simulink model "simpleObserver2withKalman"  (R2021b)
settings: Solver=ode1  StartTime=0.0  StopTime=inf  FixedStep=0.01  RelTol=1e-3
libraries: TcTargetLib x10
settings Model: Creator=ATLabor  LastModifiedBy=ATLabor
settings OptimizationCC: DefaultParameterBehavior=Inlined  LocalBlockOutputs=off
settings RTWCC: Description=TwinCAT GRT Target  SystemTargetFile=TwinCatGrt.tlc  GenCodeOnly=on  TemplateMakefile=tcgrt_msbuild.tmf  TargetLang=C++
settings STFCustomTargetCC: TargetLangStandard=C++11 (ISO)  CombineOutputUpdateFcns=on  CodeInterfacePackaging=Reusable function  CPPClassGenCompliant=on  GRTInterface=off  GenerateAllocFcn=on  SystemTargetFile=TwinCatGrt.tlc
settings GRTTargetCC: TargetLangStandard=C++11 (ISO)  ParMdlRefBuildCompliant=off  CompOptLevelCompliant=off  ConcurrentExecutionCompliant=off  MatFileLogging=off  CodeInterfacePackaging=Reusable function  GenerateAllocFcn=on  UseToolchainInfoCompliant=off  ExtModeMexFile=TcExtModeClient

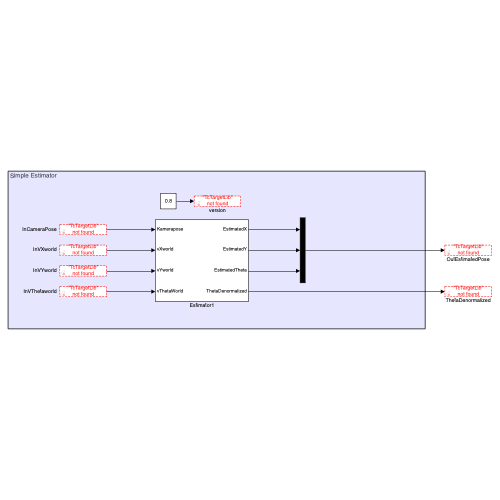
[thumbnail: Simulink's stored preview of the top-level diagram]
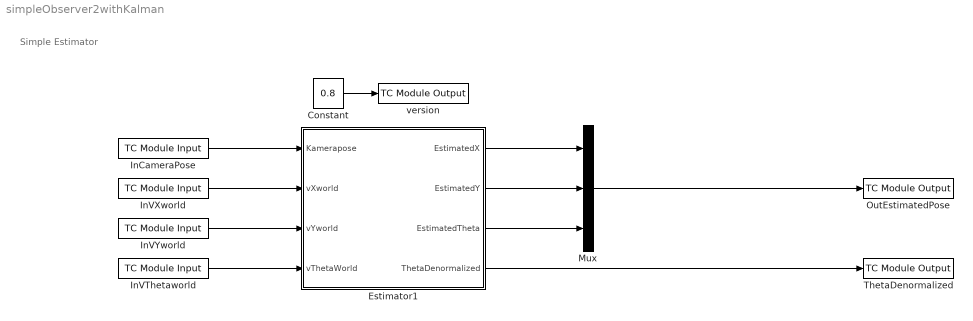
== system simpleObserver2withKalman ==
  note: Simple Estimator
  Constant : Constant  Value=0.8
  Estimator1 : Subsystem
  InCameraPose : TcTargetLib/TC Module Input  PortDataType=double  PortDim=3  Value=[0 0 0]  SampleTime=-1  CodeGenConnectType=DataArea (InputDst)  DataTypeOverride=on
      settings: SourceProductName=Beckhoff TwinCAT Target
  InVThetaworld : TcTargetLib/TC Module Input  PortDataType=double  PortDim=1  Value=0  SampleTime=-1  CodeGenConnectType=DataArea (InputDst)  DataTypeOverride=off
      settings: SourceProductName=Beckhoff TwinCAT Target
  InVXworld : TcTargetLib/TC Module Input  PortDataType=double  PortDim=1  Value=0  SampleTime=-1  CodeGenConnectType=DataArea (InputDst)  DataTypeOverride=off
      settings: SourceProductName=Beckhoff TwinCAT Target
  InVYworld : TcTargetLib/TC Module Input  PortDataType=double  PortDim=1  Value=0  SampleTime=-1  CodeGenConnectType=DataArea (InputDst)  DataTypeOverride=off
      settings: SourceProductName=Beckhoff TwinCAT Target
  Mux : Mux  Inputs=3
  OutEstimatedPose : TcTargetLib/TC Module Output  PortDataType=double  PortDim=3  SampleTime=-1  CodeGenConnectType=DataArea (OutputSrc)  DataTypeOverride=off
      settings: SourceProductName=Beckhoff TwinCAT Target
  ThetaDenormalized : TcTargetLib/TC Module Output  PortDataType=double  PortDim=1  SampleTime=-1  CodeGenConnectType=DataArea (OutputSrc)  DataTypeOverride=off
      settings: SourceProductName=Beckhoff TwinCAT Target
  version : TcTargetLib/TC Module Output  PortDataType=double  PortDim=1  SampleTime=-1  CodeGenConnectType=DataArea (OutputSrc)  DataTypeOverride=off
      settings: SourceProductName=Beckhoff TwinCAT Target
  wires:
  Mux/1 -> OutEstimatedPose/1
  InVXworld/1 -> Estimator1/2(vXworld)
  Estimator1/3(EstimatedTheta) -> Mux/3
  InCameraPose/1 -> Estimator1/1(Kamerapose)
  Estimator1/4(ThetaDenormalized) -> ThetaDenormalized/1
  Estimator1/1(EstimatedX) -> Mux/1
  InVYworld/1 -> Estimator1/3(vYworld)
  Estimator1/2(EstimatedY) -> Mux/2
  Constant/1 -> version/1
  InVThetaworld/1 -> Estimator1/4(vThetaWorld)

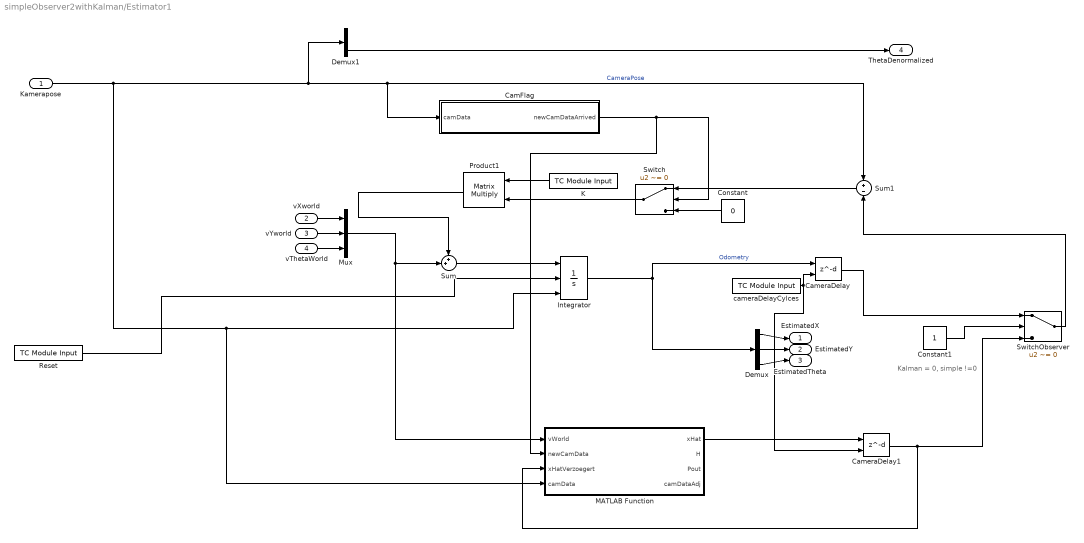
== system simpleObserver2withKalman/Estimator1 ==
  note: Kalman = 0, simple !=0
  Kamerapose : Inport  PortDimensions=3
  vXworld : Inport  Port=2
  vYworld : Inport  Port=3
  vThetaWorld : Inport  Port=4
  CamFlag : MATLAB Function  TreatAsAtomicUnit=on  SystemSampleTime=0.01
  CameraDelay : Delay  DelayLengthSource=Input port  DelayLength=14
      settings: InputPortMap=u0,p1
  CameraDelay1 : Delay  DelayLengthSource=Input port  DelayLength=14
      settings: InputPortMap=u0,p1
  Constant : Constant  Value=0
  Constant1 : Constant
  Demux : Demux  Outputs=3
  Demux1 : Demux  Outputs=3
  Integrator : Integrator  ExternalReset=rising  InitialConditionSource=external
  K : TcTargetLib/TC Module Input  PortDataType=double  PortDim=[3,3]  Value=[1,0,0;0,1,0;0,0,1]  SampleTime=-1  CodeGenConnectType=DataArea (InputDst)  DataTypeOverride=off
      settings: SourceProductName=Beckhoff TwinCAT Target
  MATLAB Function : MATLAB Function  TreatAsAtomicUnit=on
  Mux : Mux  Inputs=3
  Product1 : Product  Multiplication=Matrix(*)
  Reset : TcTargetLib/TC Module Input  PortDataType=boolean  PortDim=1  Value=0  SampleTime=-1  CodeGenConnectType=DataArea (InputDst)  DataTypeOverride=off
      settings: SourceProductName=Beckhoff TwinCAT Target
  Sum : Sum  Inputs=++|
  Sum1 : Sum  Inputs=+|-
  Switch : Switch  Criteria=u2 ~= 0  Threshold=0.5
  SwitchObserver : Switch  Criteria=u2 ~= 0
  cameraDelayCylces : TcTargetLib/TC Module Input  PortDataType=int8  PortDim=1  Value=0  SampleTime=-1  CodeGenConnectType=DataArea (InputDst)  DataTypeOverride=off
      settings: SourceProductName=Beckhoff TwinCAT Target
  EstimatedX : Outport
  EstimatedY : Outport  Port=2
  EstimatedTheta : Outport  Port=3
  ThetaDenormalized : Outport  Port=4
  wires:
  vThetaWorld/1 -> Mux/3
  vXworld/1 -> Mux/1
  Kamerapose/1 -> CamFlag/1(camData), Sum1/1, Demux1/1, MATLAB Function/4(camData), Integrator/3  "CameraPose"
  vYworld/1 -> Mux/2
  Switch/1 -> Product1/2
  Demux/2 -> EstimatedY/1
  Demux/1 -> EstimatedX/1
  Demux/3 -> EstimatedTheta/1
  Mux/1 -> MATLAB Function/1(vWorld), Sum/2
  Sum/1 -> Integrator/1
  Integrator/1 -> Demux/1, CameraDelay/1  "Odometry"
  CameraDelay/1 -> SwitchObserver/1
  Product1/1 -> Sum/1
  K/1 -> Product1/1
  Sum1/1 -> Switch/1
  Constant/1 -> Switch/3
  CamFlag/1(newCamDataArrived) -> MATLAB Function/2(newCamData), Switch/2
  Reset/1 -> Integrator/2
  cameraDelayCylces/1 -> CameraDelay/2, CameraDelay1/2
  Demux1/3 -> ThetaDenormalized/1
  SwitchObserver/1 -> Sum1/2
  MATLAB Function/1(xHat) -> CameraDelay1/1
  Constant1/1 -> SwitchObserver/2
  CameraDelay1/1 -> MATLAB Function/3(xHatVerzoegert), SwitchObserver/3

== matlab function simpleObserver2withKalman/Estimator1/MATLAB Function ==
  settings: updateMethod=DISCRETE  sampleTime=10e-3
  data: vWorld input; xHat output; newCamData input; xHatVerzoegert input; camData input; H output; Pout output; camDataAdj output
function [xHat, H, Pout, camDataAdj]= Kalman(vWorld, newCamData, xHatVerzoegert, camData)

persistent xHatOld;
persistent P;

if isempty(xHatOld)
    xHatOld = [0; 0; 0];
    xHat = xHatOld;
end

if isempty(P)
    P = zeros(3,3);
end
camDataAdj =[0; 0; 0];
%% Systemparameter
A = [1 0 0;
     0 1 0;
     0 0 1];

taskTime = 10e-3; %10ms

B = [taskTime; taskTime; taskTime];

%C = [1 1 1];
C = eye(3);

R = [0.00127820524383046    -0.00144745069148629    1.57202639633006e-06;
    -0.00144745069148629    0.0142936660651043      -2.43008878392535e-05;
    1.57202639633006e-06    -2.43008878392535e-05	2.50703907504212e-07];

% Processnoise average
% Q =[3.8635    0.4415   -0.0036;
%     0.4415    9.3899   -0.0078;
%    -0.0036   -0.0078    0.0001];

% Process noise Q like above but on diagonal values from ComvMatT3,
% ComvMatX300, CovMatY300
Q =[9.3047    0.4415   -0.0036;
    0.4415    26.0708   -0.0078;
   -0.0036   -0.0078    0.0007];

%% Prediction
xHatAp = A * xHatOld + B .* vWorld;
PAp = A * P * A' + Q;
xHat = xHatAp;
P = PAp;
%% Optimizing
%H = PAp * C' .* inv(C*PAp*C'+R);
H = PAp * inv(PAp+R);   %C nicht noetig, da Einheitsvektor

%% Correction (only when new, valid Cam-Measurement)
if newCamData
    camDataAdj = camData;
    %xHatOld = xHatVerzoegert;
    xHat = xHatAp + H * (camDataAdj - C*xHatVerzoegert);  %normal Kalman Calculation
    odomSinceCapture = xHat - xHatVerzoegert;
    xHat = xHat + odomSinceCapture; % add odometrie difference since cameraMeasurement was taken to equalize cam delay
    P = PAp - H*C*PAp;
    %P = PAp - H*PAp;
end

xHatOld = xHat;
Pout = P;

== matlab function simpleObserver2withKalman/Estimator1/CamFlag ==
  data: camData input; newCamDataArrived output
function newCamDataArrived = fcn(camData)

persistent oldCamData

if isempty(oldCamData)
    oldCamData = [0 0 0]';
end

if all(camData(1:2)) && all(camData ~= oldCamData)
    newCamDataArrived = true;
else
    newCamDataArrived = false;
    oldCamData = camData;
end
